simulink model "final_model"  (R2015b)
settings: Solver=VariableStepAuto  StartTime=0.0  StopTime=10.0  RelTol=1e-3
settings Model: Creator=MiaoshunWu  LastModifiedBy=MiaoshunWu

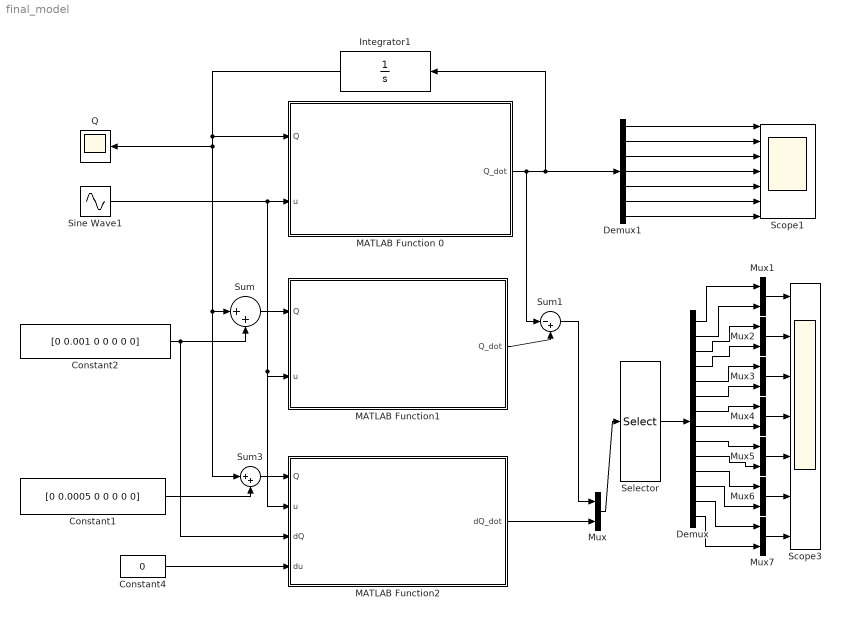
== system final_model ==
  Constant1 : Constant  Value=[0 0.0005 0 0 0 0 0]
  Constant2 : Constant  Value=[0 0.001 0 0 0 0 0]
  Constant4 : Constant  Value=0
  Demux : Demux  Outputs=14
  Demux1 : Demux  Outputs=7
  Integrator1 : Integrator  InitialCondition=[0;0;0;0;0;0;0;]
  MATLAB Function 0 : MATLAB Function  TreatAsAtomicUnit=on
  MATLAB Function1 : MATLAB Function  TreatAsAtomicUnit=on
  MATLAB Function2 : MATLAB Function  TreatAsAtomicUnit=on
  Mux{,1..7} (8 alike) : Mux  Inputs=2
  Q : Scope
  Scope1 : Scope  NumInputPorts=7
  Scope3 : Scope  NumInputPorts=7
  Selector : Selector  InputPortWidth=14  IndexOptions=Index vector (dialog)  Indices=[1 8 2 9 3 10 4 11 5 12 6 13 7 14]  OutputSizes=1
  Sine Wave1 : Sin  SampleTime=0
  Sum : Sum  Inputs=|++
  Sum1 : Sum  Inputs=|-+
  Sum3 : Sum  Inputs=|++
  wires:
  MATLAB Function 0/1(Q_dot) -> Demux1/1, Integrator1/1, Sum1/1
  Sine Wave1/1 -> MATLAB Function2/2(u), MATLAB Function1/2(u), MATLAB Function 0/2(u)
  Sum/1 -> MATLAB Function1/1(Q)
  MATLAB Function1/1(Q_dot) -> Sum1/2
  Integrator1/1 -> MATLAB Function 0/1(Q), Sum/1, Sum3/1, Q/1
  MATLAB Function2/1(dQ_dot) -> Mux/2
  Constant2/1 -> Sum/2, MATLAB Function2/3(dQ)
  Constant1/1 -> Sum3/2
  Sum3/1 -> MATLAB Function2/1(Q)
  Constant4/1 -> MATLAB Function2/4(du)
  Mux/1 -> Selector/1
  Selector/1 -> Demux/1
  Demux/1 -> Mux1/1
  Mux2/1 -> Scope3/2
  Mux3/1 -> Scope3/3
  Demux/7 -> Mux4/1
  Demux/8 -> Mux4/2
  Mux1/1 -> Scope3/1
  Mux4/1 -> Scope3/4
  Demux/6 -> Mux3/2
  Demux/5 -> Mux3/1
  Demux/4 -> Mux2/2
  Demux/3 -> Mux2/1
  Demux/2 -> Mux1/2
  Demux/9 -> Mux5/1
  Demux/10 -> Mux5/2
  Demux/11 -> Mux6/1
  Demux/12 -> Mux6/2
  Demux/13 -> Mux7/1
  Demux/14 -> Mux7/2
  Mux5/1 -> Scope3/5
  Mux6/1 -> Scope3/6
  Mux7/1 -> Scope3/7
  Demux1/1 -> Scope1/1
  Demux1/2 -> Scope1/2
  Demux1/3 -> Scope1/3
  Demux1/4 -> Scope1/4
  Demux1/5 -> Scope1/5
  Demux1/6 -> Scope1/6
  Demux1/7 -> Scope1/7
  Sum1/1 -> Mux/1

== matlab function final_model/MATLAB Function 0 ==
  data: Q_dot output; Q input; u input
function Q_dot  = DIP_Model(Q,u)
%{
%Description: Double inverted pendulum model
%Purpose: Simulates the double inverted pendulum through its mathematical 
%         dynamic model            
%Input Parameters: State space "Q", control input "u"
%Output Parameters: Derivative state space "Q_dot"
%Author: A. Arreortua
%**************************************************************************
%}
%% Definition of constants
% gravity acceleration
g = 9.81; % [m/s^2]
a1=0.085; %Distance between pivot and center of mass of pendulum1 [m]
a2=0.157; %Distance between pivot and center of mass of pendulum2 [m]
l1= 0.170; %Length of pendulum1 [m]
l2= 0.314;  %Length of pendulum2 [m]
m1=0.162; %Mass of pendulum1 [kg]
m2=0.203; %Mass of pendulum2 [kg]
J1 = (m1*l1^2)/12;    %Inertia of pendulum1 around the joint [kg m^2]
J2 = (m2*l2^2)/12;    %Inertia of pendulum2 around the joint [kg m^2]
% Model of motor behaviour: PT1 tau
T1 = 0.0395; % [s]
%Dinamic model constants
h2 = m1*a1+m2*l1;
h3 = m2*a2;
h4 = m1*a1^2+m2*l1^2+J1;
h5 = m2*a2*l1;
h6 = m2*a2^2+J2;
h7 = m1*a1*g + m2*l1*g;
h8 = m2*a2*g;

Q0=Q(1); 
Q1=Q(2);
Q2=Q(3);
Q3=Q(4); 
Q5=Q(6);

det = (h4 * h6 - h5 * h5 * cos(Q2 - Q3) * cos(Q2 - Q3));
M11inv= [h6/det ,-h5*cos(Q2-Q3)/det ; -h5*cos(Q2-Q3)/det ,h4/det];
M12 = [h2*cos(Q2); h3*cos(Q3)];
C1 = [h5*(Q1^2)*sin(Q2-Q3); -h5*(Q0^2)*sin(Q2-Q3)];
G1 = [-h7*sin(Q2); -h8*sin(Q3)];


%% Dynamic equations
x_2dot = ((u-Q5)/T1);  %%% x_2dot=
Theta_2dot = -M11inv*(M12* x_2dot + C1 + G1);
Q_dot = [Theta_2dot;Q0;Q1;Q5;x_2dot;u*u];

== matlab function final_model/MATLAB Function1 ==
  data: Q_dot output; Q input; u input
function Q_dot = DIP_Model(Q,u)
% gravity acceleration
g = 9.81; % [m/s^2]
a1=0.085; %Distance between pivot and center of mass of pendulum1 [m]
a2=0.157; %Distance between pivot and center of mass of pendulum2 [m]
l1= 0.170; %Length of pendulum1 [m]
l2= 0.314;  %Length of pendulum2 [m]
m1=0.162; %Mass of pendulum1 [kg]
m2=0.203; %Mass of pendulum2 [kg]
J1 = (m1*l1^2)/12;    %Inertia of pendulum1 around the joint [kg m^2]
J2 = (m2*l2^2)/12;    %Inertia of pendulum2 around the joint [kg m^2]
% Model of motor behaviour: PT1 tau
T1 = 0.0395; % [s]
%Dinamic model constants
h2 = m1*a1+m2*l1;
h3 = m2*a2;
h4 = m1*a1^2+m2*l1^2+J1;
h5 = m2*a2*l1;
h6 = m2*a2^2+J2;
h7 = m1*a1*g + m2*l1*g;
h8 = m2*a2*g;

Q0=Q(1); 
Q1=Q(2);
Q2=Q(3);
Q3=Q(4); 
Q5=Q(6);

det = (h4* h6 - h5 * h5 * cos(Q2 - Q3) * cos(Q2 - Q3));
M11inv= [h6/det ,-h5*cos(Q2-Q3)/det ; -h5*cos(Q2-Q3)/det ,h4/det];
M12 = [h2*cos(Q2); h3*cos(Q3)];
C1 = [h5*(Q1^2)*sin(Q2-Q3); -h5*(Q0^2)*sin(Q2-Q3)];
G1 = [-h7*sin(Q2); -h8*sin(Q3)];


x05 = ((u-Q5)/T1);
N1 = (M12(1)*x05 + C1(1) + G1(1));
N2 = (M12(2)*x05 + C1(2) + G1(2));
x00 = -M11inv(1,1) *N1 +(- M11inv(1,2) * N2 );
x01 = -M11inv(2,1) *N1 +(- M11inv(2,2) * N2 );
x02 = Q0;
x03 = Q1;
x04 = Q5;
x06 = u * u;
dx=[x00;x01;x02;x03;x04;x05;x06];
Q_dot=dx;
end

== matlab function final_model/MATLAB Function2 ==
  data: dQ_dot output; Q input; u input; dQ input; du input
function dQ_dot  = DIP_Model(Q,u,dQ,du)
%{
%Description: Double inverted pendulum model
%Purpose: Simulates the double inverted pendulum through its mathematical 
%         dynamic model            
%Input Parameters: State space "Q", control input "u"
%Output Parameters: Derivative state space "Q_dot"
%Author: A. Arreortua
%**************************************************************************
%}
%% Definition of constants
g = 9.81; % [m/s^2]
a1=0.085; %Distance between pivot and center of mass of pendulum1 [m]
a2=0.157; %Distance between pivot and center of mass of pendulum2 [m]
l1= 0.170; %Length of pendulum1 [m]
l2= 0.314;  %Length of pendulum2 [m]
m1=0.162; %Mass of pendulum1 [kg]
m2=0.203; %Mass of pendulum2 [kg]
J1 = (m1*l1^2)/12;    %Inertia of pendulum1 around the joint [kg m^2]
J2 = (m2*l2^2)/12;    %Inertia of pendulum2 around the joint [kg m^2]
% Model of motor behaviour: PT1 tau
T1 = 0.0395; % [s]
%Dinamic model constants
h2 = m1*a1+m2*l1;
h3 = m2*a2;
h4 = m1*a1^2+m2*l1^2+J1;
h5 = m2*a2*l1;
h6 = m2*a2^2+J2;
h7 = m1*a1*g + m2*l1*g;
h8 = m2*a2*g;

x0=Q(1); 
x1=Q(2);
x2=Q(3);
x3=Q(4); 
x5=Q(6);
def=(h4 * h6 - h5 * h5 * cos(x2 - x3)* cos(x2 - x3));
P=h5 * h5 * sin(2*(x2 - x3));
%x00 = -M11inv(1,1) *N1 +(- M11inv(1,2) * N2 );
%x05 = ((u-x5)/T1);
%N1 = (M12(1)*x05 + C1(1) + G1(1));
%N2 = (M12(2)*x05 + C1(2) + G1(2));

%x00 = -M11inv(1,1) *N1 +(- M11inv(1,2) * N2 );
s00 = -(2 * x0 * h5 * h5 * cos(x2 - x3) * sin(x2 - x3)) / def;
s01=  -(2 * x1 * h5 * h6 * sin(x2 - x3)) / def;
s02= h2*h6*(u-x5)*(sin(x2)*def+P*cos(x2))/(T1*def*def) - h5*h6*x1*x1*(cos(x2-x3)*def-P*sin(x2-x3))/(def*def) + h6*h7*(cos(x2)*def-P*sin(x2))/(def*def)-h3*h5*(u-x5)*cos(x3)*(sin(x2-x3)*def+P*cos(x2-x3))/(def*def*T1)- h5*h5*x0*x0*(2*cos(2*(x2-x3))*def-P*sin(2*(x2-x3)))/(2*def*def)+h5*h8*sin(x3)*(sin(x2-x3)*def+P*cos(x2-x3))/(def*def);
s03= -h2*h6*cos(x2)*(u-x5)*P/(T1*def*def) - h6*h5*x1*x1*(-cos(x2-x3)*def+P*sin(x2-x3))/(def*def) + h6*h7*sin(x2)*P/(def*def) + h5*h3*(u-x5)*(sin(x2-2*x3)*def+P*cos(x2-x3)*cos(x3))/(T1*def*def) - h5*h5*x0*x0*(-2*cos(2*(x2-x3))*def+P*sin(2*(x2-x3)))/(2*def*def) - h8*h5*(cos(x2-2*x3)*def+P*cos(x2-x3)*sin(x3))/(def*def);
s04 = 0;
s05 = ( h2 * h6 * cos(x2)- h3 * h5 * cos(x3) * cos(x2 - x3)) / (T1 * (def));
s06 = -(h2 * h6 * cos(x2)- h3 * h5 * cos(x3) * cos(x2 - x3)) / (T1 * (def));
ddx0 = dQ(1)*s00+dQ(2)*s01+dQ(3)*s02+dQ(4)*s03+dQ(5)*s04+dQ(6)*s05+du*s06;


%x01 = -M11inv(2,1) *N1 +(- M11inv(2,2) * N2 );
s10 = (2 * x0 * h4 * h5 * sin(x2 - x3)) / def;
s11 = (2 * x1 * h5 * h5 * cos(x2 - x3) * sin(x2 - x3)) /def;
s12 = h5*h2*(u-x5)*((-cos(x2-x3)*sin(x2)-sin(x2-x3)*cos(x2))*def-P*cos(x2)*cos(x2-x3))/(T1*def*def)  +   h5*h5*x1*x1*(2*cos(2*(x2-x3))*def-P*sin(2*(x2-x3)))/(2*def*def)   - h5*h7*(cos(2*x2-x3)*def-P*cos(x2-x3)*sin(x2))/(def*def) + h4*h3*(u-x5)*P*cos(x3)/(T1*def*def) + h5*h4*x0*x0*(cos(x2-x3)*def-P*sin(x2-x3))/(def*def) - h4*h8*sin(x3)*P/(def*def);		
s13=  h2*h5*(u-x5)*cos(x2)*(sin(x2-x3)*def+P*cos(x2-x3))/(def*def*T1) + h5*h5*x1*x1*(-2*cos(2*(x2-x3))*def+P*sin(2*(x2-x3)))/(2*def*def) - h5*h7*sin(x2)*(sin(x2-x3)*def+P*cos(x2-x3))/(def*def) - h4*h3*(u-x5)*(-sin(x3)*def+P*cos(x3))/(T1*def*def) + h4*h5*x0*x0*(-cos(x2-x3)*def+P*sin(x2-x3))/(def*def) +  h4*h8*(cos(x3)*def+P*sin(x3))/(def*def);
s14 = 0;
s15 =  ((h3 * h4 * cos(x3)) - (h2 * h5 * cos(x2) * cos(x2 - x3))) / (T1 * (h4 * h6 - h5 * h5 * cos(x2 - x3) * cos(x2 - x3)));
s16 = -((h3 * h4 * cos(x3)) - (h2 * h5 * cos(x2) * cos(x2 - x3))) / (T1 * (h4 * h6 - h5 * h5 * cos(x2 - x3) * cos(x2 - x3)));
ddx1=dQ(1)*s10+dQ(2)*s11+dQ(3)*s12+dQ(4)*s13+dQ(5)*s14+dQ(6)*s15+du*s16;



ddx2=dQ(1);
%s(2, x_indexode(0)) = 1;
%s(2, x_indexode(1)) = 0;
%s(2, x_indexode(2)) = 0;
%s(2, x_indexode(3)) = 0;
%s(2, x_indexode(4)) = 0;
%s(2, x_indexode(5)) = 0;
%s(2, u_indexode(0)) = 0;

ddx3=dQ(2);
%s(3, x_indexode(0)) = 0;
%s(3, x_indexode(1)) = 1;
%s(3, x_indexode(2)) = 0;
%s(3, x_indexode(3)) = 0;
%s(3, x_indexode(4)) = 0;
%s(3, x_indexode(5)) = 0;
%s(3, u_indexode(0)) = 0;

 ddx4=dQ(6);
%s(4, x_indexode(0)) = 0;
%s(4, x_indexode(1)) = 0;
%s(4, x_indexode(2)) = 0;
%s(4, x_indexode(3)) = 0;
%s(4, x_indexode(4)) = 0;
%s(4, x_indexode(5)) = 1;
%s(4, u_indexode(0)) = 0;

 ddx5=(du-dQ(6))/ T1;
%s(5, x_indexode(0)) = 0;
%s(5, x_indexode(1)) = 0;
%s(5, x_indexode(2)) = 0;
%s(5, x_indexode(3)) = 0;
%s(5, x_indexode(4)) = 0;
%s(5, x_indexode(5)) = -1 / T1;
%s(5, u_indexode(0)) = 1 / T1;
 ddx6 =(du* du);
%s(6, x_indexode(0)) = 0;     //!!!!!
%s(6, x_indexode(1)) = 0;
%s(6, x_indexode(2)) = 0;
%s(6, x_indexode(3)) = 0;
%s(6, x_indexode(4)) = 0;
%s(6, x_indexode(5)) = 0;
%s(6, u_indexode(0)) = 2 * u;

%% Dynamic equations
dQ_dot=[ddx0;ddx1;ddx2;ddx3;ddx4;ddx5;ddx6];
